simulink model "nid_sl"  (Simulink 10.0)
settings: Solver=FixedStepDiscrete  StartTime=0.0  StopTime=inf  RelTol=1e-3  EnableMultiTasking=on
StartFcn:
  | h = add_exec_event_listener('nid_sl/NID Image', 'PreOutputs',@Image_out);
libraries: nid_lib x3
settings Model: Creator=tchikama  LastModifiedBy=bhisma
settings DataIOCC: LimitDataPoints=on  SignalLoggingSaveFormat=ModelDataLogs  SaveOutput=off
settings OptimizationCC: ExpressionDepthLimit=2147483647  SimCompilerOptimization=on
settings DebuggingCC: SolverPrmCheckMsg=warning  FcnCallInpInsideContextMsg=warning  StateNameClashWarn=warning
settings HardwareCC: ProdIntDivRoundTo=Zero  ProdEndianess=LittleEndian  ProdHWDeviceType=Generic->32-bit x86 compatible
settings RTWCC: RTWCompilerOptimization=on
settings CodeAppCC: MaxIdLength=95
settings GRTTargetCC: GeneratePreprocessorConditionals=Disable all
settings ConfigComp: CovExternalEMLEnable=off

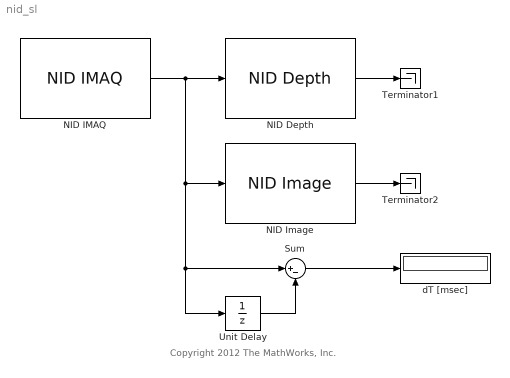
== system nid_sl ==
  note: Copyright 2012 The MathWorks, Inc.
  NID Depth : nid_lib/NID Depth  depthOutput=Depth  conv_XYZ_RW=off  viewer=off
  NID IMAQ : nid_lib/NID IMAQ  imaq_depth=on  imaq_motion=off  imaq_image=on  view_point=off  imaq_skeleton=off  imaq_ir=off  mirror_image=off  imaq_sample_time=1/30  res_fps=VGA (640x480): 30 FPS  needPsiPose=off  angle_input=off  angle=0  angle_read=off  near_mode=off  seated_mode=off  skeleton_smooth=[0.5 0.5 0.5 0.05 0.04]  infer_skeleton=on
  NID Image : nid_lib/NID Image  imageOutput=RGB
  Sum : Sum  Inputs=|+-
  Terminator1 : Terminator
  Terminator2 : Terminator
  Unit Delay : UnitDelay  SampleTime=-1
  dT [msec] : Display
  wires:
  NID Depth/1 -> Terminator1/1
  NID IMAQ/1 -> NID Depth/1, Sum/1, Unit Delay/1, NID Image/1
  Sum/1 -> dT [msec]/1
  NID Image/1 -> Terminator2/1
  Unit Delay/1 -> Sum/2
